simulink model "Read_optitrack"  (R2020a)
settings: Solver=FixedStepAuto  StartTime=0.0  StopTime=inf  RelTol=1e-3
model workspace (MAT data in the model file):
  SL_ROS_VariableLengthArrays_MaxSizes.CommonInfo.ArrayTruncateAction = 'EmitWarning'
  SL_ROS_VariableLengthArrays_MaxSizes.MsgTypeMap = containers.Map
  SL_ROS_VariableLengthArrays_MaxSizes.MsgTypeMap.serialization.keys = {'sensor_msgs/CompressedImage', 'sensor_msgs/LaserScan'}
  SL_ROS_VariableLengthArrays_MaxSizes.MsgTypeMap.serialization.values{1}(1).PropertyName = 'Data'
  SL_ROS_VariableLengthArrays_MaxSizes.MsgTypeMap.serialization.values{1}(1).DataType = 'uint8'
  SL_ROS_VariableLengthArrays_MaxSizes.MsgTypeMap.serialization.values{1}(1).MaxLength = 200000
  SL_ROS_VariableLengthArrays_MaxSizes.MsgTypeMap.serialization.values{1}(2).PropertyName = 'Format'
  SL_ROS_VariableLengthArrays_MaxSizes.MsgTypeMap.serialization.values{1}(2).DataType = 'uint8'
  SL_ROS_VariableLengthArrays_MaxSizes.MsgTypeMap.serialization.values{1}(2).MaxLength = 128
  SL_ROS_VariableLengthArrays_MaxSizes.MsgTypeMap.serialization.values{2}(1).PropertyName = 'Intensities'
  SL_ROS_VariableLengthArrays_MaxSizes.MsgTypeMap.serialization.values{2}(1).DataType = 'single'
  SL_ROS_VariableLengthArrays_MaxSizes.MsgTypeMap.serialization.values{2}(1).MaxLength = 360
  SL_ROS_VariableLengthArrays_MaxSizes.MsgTypeMap.serialization.values{2}(2).PropertyName = 'Ranges'
  SL_ROS_VariableLengthArrays_MaxSizes.MsgTypeMap.serialization.values{2}(2).DataType = 'single'
  SL_ROS_VariableLengthArrays_MaxSizes.MsgTypeMap.serialization.values{2}(2).MaxLength = 360
  SL_ROS_VariableLengthArrays_MaxSizes.MsgTypeMap.serialization.uniformity = 0
  SL_ROS_VariableLengthArrays_MaxSizes.MsgTypeMap.serialization.keyType = 'char'
  SL_ROS_VariableLengthArrays_MaxSizes.MsgTypeMap.serialization.valueType = 'any'
undefined symbols (not defined in the file): Angular, Linear
libraries: robotlib x3, simulink_extras x2, realtime_pacer_lib x2, vrlib x1, simulink x1, sharedtransform x1
settings Model: Creator=20195009  LastModifiedBy=TruckLabPC2
settings OptimizationCC: EnhancedBackFolding=on  PassReuseOutputArgsAs=Individual arguments  ZeroExternalMemoryAtStartup=off  ZeroInternalMemoryAtStartup=off  MaxStackSize=64  OptimizeBlockOrder=speed  DifferentSizesBufferReuse=on  OptimizationCustomize=off  EfficientTunableParamExpr=on
settings DebuggingCC: ParameterTunabilityLossMsg=error  SFMachineParentedDataDiag=error
settings HardwareCC: ProdBitPerPointer=32  ProdBitPerSizeT=32  ProdBitPerPtrDiffT=32  ProdLargestAtomicFloat=None  ProdIntDivRoundTo=Undefined  ProdEndianess=Unspecified  ProdWordSize=32  ProdHWDeviceType=Generic->Unspecified (assume 32-bit Generic)
settings SFSimCC: MATLABDynamicMemAlloc=off
settings RTWCC: SystemTargetFile=ert.tlc  HardwareBoard=Robot Operating System (ROS)  TemplateMakefile=ert_default_tmf  Toolchain=Catkin  TargetLang=C++
settings CodeAppCC: ForceParamTrailComments=on  IgnoreCustomStorageClasses=off  OperatorAnnotations=on  SimulinkDataObjDesc=on  SFDataObjDesc=on  InsertBlockDesc=on

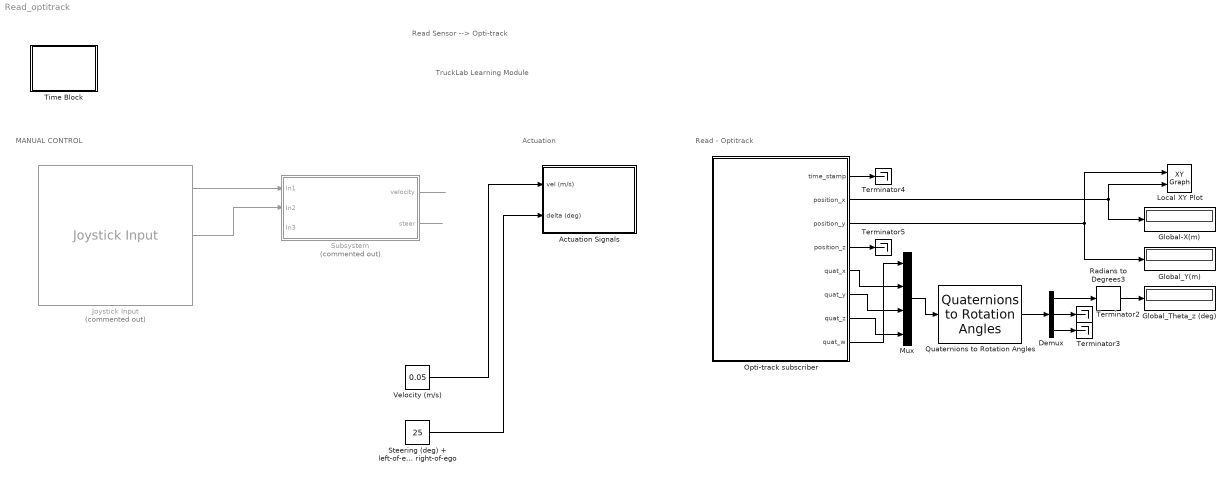
== system Read_optitrack ==
  note: Read - Optitrack
  note: MANUAL CONTROL
  note: TruckLab Learning Module
  note: Read Sensor --> Opti-track
  note: Actuation
  Actuation Signals : Subsystem
  Demux : Demux  Outputs=3
  Global-X(m) : Display
  Global_Theta_z (deg) : Display
  Global_Y(m) : Display
  Joystick Input : vrlib/Joystick Input  Commented=on  joyid=1  adjustports=on  forcefeed=off
  Local XY Plot : simulink/Sinks/XY Graph  xmin=0  xmax=6  ymin=0  ymax=6  st=-1
  Mux : Mux
  Opti-track subscriber : Subsystem
  Quaternions to Rotation Angles : sharedtransform/Quaternions to Rotation Angles  rotationOrder=ZXY  aMode=aMode
      settings: SourceProductBaseCode=AE,PW,MT,VE,VP
  Radians to Degrees3 : simulink_extras/Transformations/Radians to Degrees
  Steering (deg) + left-of-ego - right-of-ego : Constant  Value=25
  Subsystem : Subsystem  Commented=on
  Terminator{2..5} (4 alike) : Terminator
  Time Block : Subsystem
  Velocity (m/s) : Constant  Value=0.05
  wires:
  Opti-track subscriber/3(position_y) -> Global_Y(m)/1, Local XY Plot/1
  Opti-track subscriber/2(position_x) -> Global-X(m)/1, Local XY Plot/2
  Mux/1 -> Quaternions to Rotation Angles/1
  Quaternions to Rotation Angles/1 -> Demux/1
  Demux/1 -> Radians to Degrees3/1
  Radians to Degrees3/1 -> Global_Theta_z (deg)/1
  Demux/2 -> Terminator2/1
  Demux/3 -> Terminator3/1
  Opti-track subscriber/5(quat_x) -> Mux/2
  Opti-track subscriber/6(quat_y) -> Mux/3
  Opti-track subscriber/7(quat_z) -> Mux/4
  Opti-track subscriber/8(quat_w) -> Mux/1
  Opti-track subscriber/1(time_stamp) -> Terminator4/1
  Opti-track subscriber/4(position_z) -> Terminator5/1
  ? -> Subsystem/3(In3)
  Steering (deg) + left-of-ego - right-of-ego/1 -> Actuation Signals/2(delta (deg))
  Subsystem/1(velocity) -> ?
  Subsystem/2(steer) -> ?
  Joystick Input/2 -> Subsystem/2(In2)
  Velocity (m/s)/1 -> Actuation Signals/1(vel (m/s))
  Joystick Input/1 -> Subsystem/1(In1)

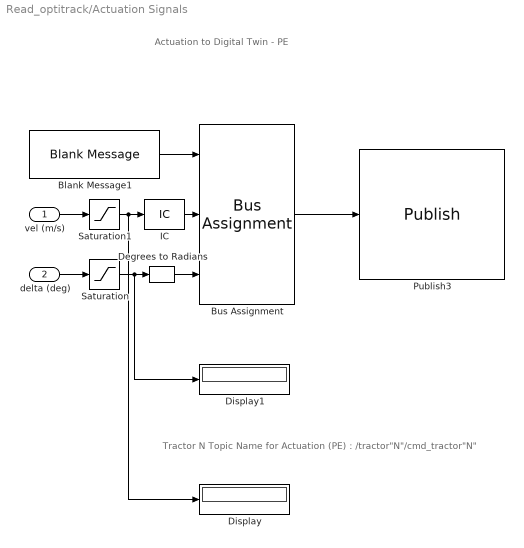
== system Read_optitrack/Actuation Signals ==
  note: Tractor N Topic Name for Actuation (PE) : /tractor"N"/cmd_tractor"N"
  note: Actuation to Digital Twin - PE
  vel (m/s) : Inport
  delta (deg) : Inport  Port=2
  Blank Message1 : robotlib/Blank Message  messageClass=Message  entityType=geometry_msgs/Twist  messageType=geometry_msgs/Twist  SampleTime=0.01
  Bus Assignment : BusAssignment  DialogController=Simulink.DDGSource_BusAssignment  AssignedSignals=Linear.X,Angular.Z
  Degrees to Radians : simulink_extras/Transformations/Degrees to Radians
  Display : Display
  Display1 : Display
  IC : InitialCondition  Value=0
  Publish3 : robotlib/Publish  topicSource=Select from ROS network  topic=/tractor1/cmd_tractor1  messageType=geometry_msgs/Twist  messageQueueLength=1
      link override SinkBlock: ROSTopic=/cmd_vel  ROSMessageType=geometry_msgs/Twist  SLBusName=SL_Bus_TruckLab_MannualDrivingROS1_geometry_msgs_Twist  ModelName=TruckLab_MannualDrivingROS1  BlockId=Pub_TruckLab_MannualDrivingROS1_402
  Saturation : Saturate  UpperLimit=25  LowerLimit=-25
  Saturation1 : Saturate  UpperLimit=0.28  LowerLimit=-0.28
  wires:
  vel (m/s)/1 -> Saturation1/1
  IC/1 -> Bus Assignment/2
  Bus Assignment/1 -> Publish3/1
  Degrees to Radians/1 -> Bus Assignment/3
  Blank Message1/1 -> Bus Assignment/1
  delta (deg)/1 -> Saturation/1
  Saturation/1 -> Display1/1, Degrees to Radians/1
  Saturation1/1 -> Display/1, IC/1

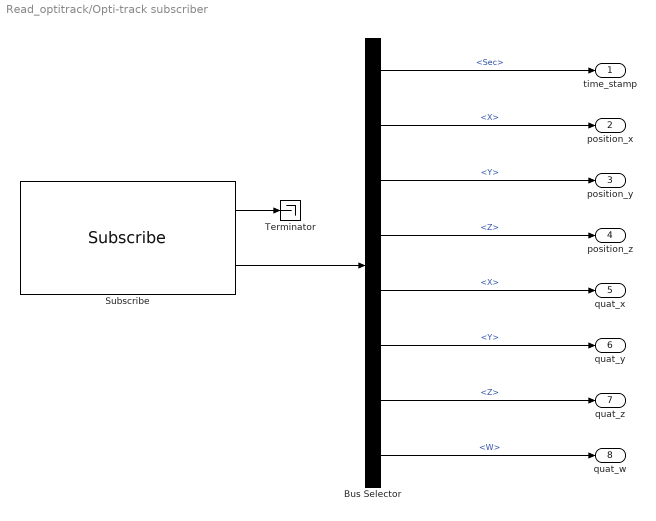
== system Read_optitrack/Opti-track subscriber ==
  Bus Selector : BusSelector  OutputSignals=Header.Stamp.Sec,Pose.Position.X,Pose.Position.Y,Pose.Position.Z,Pose.Orientation.X,Pose.Orientation.Y,Pose.Orientation.Z,Pose.Orientation.W
  Subscribe : robotlib/Subscribe  topicSource=Select from ROS network  topic=/DC_1/TRACTOR_1/optitrack  messageType=geometry_msgs/PoseStamped  sampleTime=-1  messageQueueLength=1
  Terminator : Terminator
  time_stamp : Outport
  position_x : Outport  Port=2
  position_y : Outport  Port=3
  position_z : Outport  Port=4
  quat_x : Outport  Port=5
  quat_y : Outport  Port=6
  quat_z : Outport  Port=7
  quat_w : Outport  Port=8
  wires:
  Subscribe/1 -> Terminator/1
  Subscribe/2 -> Bus Selector/1
  Bus Selector/1 -> time_stamp/1  "<Sec>"
  Bus Selector/2 -> position_x/1  "<X>"
  Bus Selector/3 -> position_y/1  "<Y>"
  Bus Selector/4 -> position_z/1  "<Z>"
  Bus Selector/5 -> quat_x/1  "<X>"
  Bus Selector/6 -> quat_y/1  "<Y>"
  Bus Selector/7 -> quat_z/1  "<Z>"
  Bus Selector/8 -> quat_w/1  "<W>"

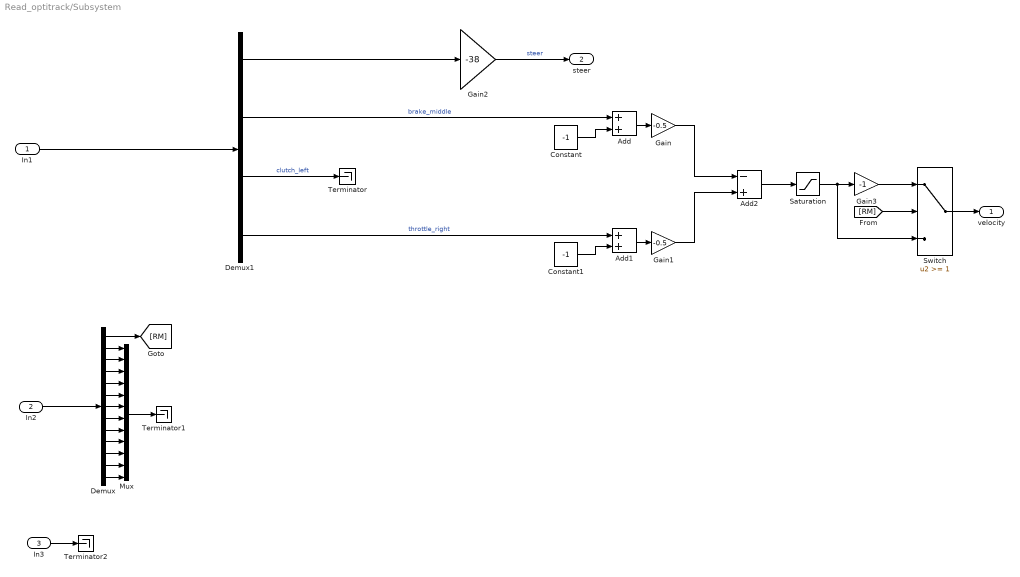
== system Read_optitrack/Subsystem ==
  In1 : Inport
  In2 : Inport  Port=2
  In3 : Inport  Port=3
  Add : Sum
  Add1 : Sum
  Add2 : Sum  Inputs=-+
  Constant : Constant  Value=-1
  Constant1 : Constant  Value=-1
  Demux : Demux  Outputs=13
  Demux1 : Demux
  Gain : Gain  Gain=-0.5
  Gain1 : Gain  Gain=-0.5
  Gain2 : Gain  Gain=-38
  Gain3 : Gain  Gain=-1
  Mux : Mux  Inputs=12
  Saturation : Saturate  UpperLimit=5  LowerLimit=0
  Switch : Switch  Threshold=1
  Terminator : Terminator
  Terminator1 : Terminator
  Terminator2 : Terminator
  velocity : Outport
  steer : Outport  Port=2
  wires:
  [RM] -> Switch/2
  Gain3/1 -> Switch/1
  Demux1/4 -> Add1/1  "throttle_right"
  Switch/1 -> velocity/1
  Demux/1 -> [RM]
  Demux1/3 -> Terminator/1  "clutch_left"
  Mux/1 -> Terminator1/1
  In1/1 -> Demux1/1
  In2/1 -> Demux/1
  Demux/6 -> Mux/5
  Demux1/1 -> Gain2/1
  Demux/8 -> Mux/7
  In3/1 -> Terminator2/1
  Constant1/1 -> Add1/2
  Constant/1 -> Add/2
  Demux/9 -> Mux/8
  Demux/12 -> Mux/11
  Demux/5 -> Mux/4
  Demux/3 -> Mux/2
  Demux/10 -> Mux/9
  Gain2/1 -> steer/1  "steer"
  Gain1/1 -> Add2/2
  Add/1 -> Gain/1
  Demux1/2 -> Add/1  "brake_middle"
  Add2/1 -> Saturation/1
  Demux/7 -> Mux/6
  Demux/11 -> Mux/10
  Saturation/1 -> Switch/3, Gain3/1
  Demux/2 -> Mux/1
  Add1/1 -> Gain1/1
  Gain/1 -> Add2/1
  Demux/13 -> Mux/12
  Demux/4 -> Mux/3

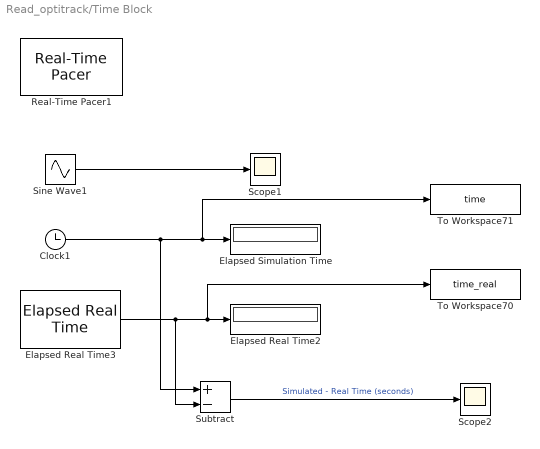
== system Read_optitrack/Time Block ==
  Clock1 : Clock
  Elapsed Real Time2 : Display
      settings: Decimation=2
  Elapsed Real Time3 : realtime_pacer_lib/Elapsed Real Time
  Elapsed Simulation Time : Display
      settings: Decimation=2
  Real-Time Pacer1 : realtime_pacer_lib/Real-Time Pacer  simTimePerRealTime=1
  Scope1 : Scope
  Scope2 : Scope
  Sine Wave1 : Sin  Frequency=2*pi*0.5  SampleTime=0
  Subtract : Sum  Inputs=+-
  To Workspace70 : ToWorkspace  VariableName=time_real  SampleTime=-1
  To Workspace71 : ToWorkspace  VariableName=time  SampleTime=-1
  wires:
  Subtract/1 -> Scope2/1  "Simulated - Real Time (seconds)"
  Elapsed Real Time3/1 -> Elapsed Real Time2/1, To Workspace70/1, Subtract/2
  Sine Wave1/1 -> Scope1/1
  Clock1/1 -> Subtract/1, Elapsed Simulation Time/1, To Workspace71/1
